simulink model "lab1_system2"  (R2024a)
settings: Solver=VariableStepAuto  StartTime=0.0  StopTime=10.0  RelTol=1e-3
undefined symbols (not defined in the file): a0, a1, a2, b0, b1, b2
settings Model: Creator=alexivanov  LastModifiedBy=alexivanov

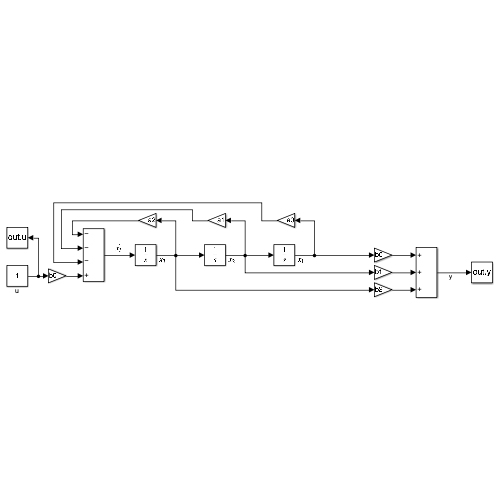
[thumbnail: Simulink's stored preview of the top-level diagram]
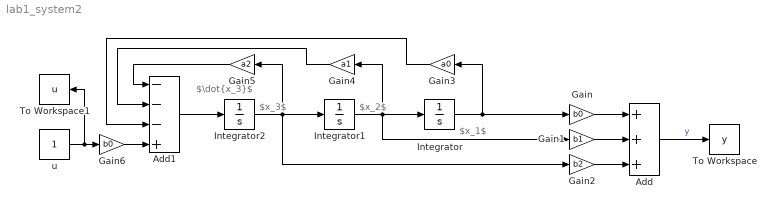
== system lab1_system2 ==
  note: $x_1$
  note: $x_2$
  note: $x_3$
  note: $\dot{x_3}$
  Add : Sum  Inputs=+++
  Add1 : Sum  Inputs=---+
  Gain : Gain  Gain=b0
  Gain1 : Gain  Gain=b1
  Gain2 : Gain  Gain=b2
  Gain3 : Gain  Gain=a0
  Gain4 : Gain  Gain=a1
  Gain5 : Gain  Gain=a2
  Gain6 : Gain  Gain=b0
  Integrator : Integrator
  Integrator1 : Integrator
  Integrator2 : Integrator
  To Workspace : ToWorkspace  VariableName=y  SaveFormat=Timeseries  SampleTime=-1
  To Workspace1 : ToWorkspace  VariableName=u  SaveFormat=Timeseries  SampleTime=-1
  u : Constant  SampleTime=0
  wires:
  Gain2/1 -> Add/3
  Gain1/1 -> Add/2
  Gain/1 -> Add/1
  Add/1 -> To Workspace/1  "y"
  Integrator1/1 -> Integrator/1, Gain4/1, Gain1/1
  Integrator2/1 -> Gain5/1, Integrator1/1, Gain2/1
  Integrator/1 -> Gain3/1, Gain/1
  Add1/1 -> Integrator2/1
  Gain5/1 -> Add1/1
  Gain4/1 -> Add1/2
  Gain3/1 -> Add1/3
  Gain6/1 -> Add1/4
  u/1 -> To Workspace1/1, Gain6/1
